simulink model "MSDR_v1"  (R2018a)
settings: Solver=ode23tb  StartTime=0.0  StopTime=50000  RelTol=1e-3
values from neighbouring files (symbols this model uses):
  a_f = -3.22E-5    (= -3.22e-05)    [MSDR_parameters.m]
  a_g = +2.35E-5    (= 2.35e-05)    [MSDR_parameters.m]
  beta = [0.000223, 0.001457, 0.001307, 0.002628, 0.000766, 0.000280]    [MSDR_parameters.m]
  beta_t = sum(beta)    [MSDR_parameters.m]
  Cp_s_shx = 1549.12e-6    (= 0.00154912)    [MSDR_parameters.m]
  Cst = 10    [MSDR_parameters.m]
  dLb = 0    [MSDR_parameters.m]
  dLs = 0    [MSDR_parameters.m]
  dLsc = 0    [MSDR_parameters.m]
  gamma_I = 5.1135e-2    (= 0.051135)    [MSDR_parameters.m]
  gamma_Xe = 1.1628e-2    (= 0.011628)    [MSDR_parameters.m]
  hA_fg = [h_fg*A_fg/2, h_fg*A_fg/2]    [MSDR_parameters.m]
  hA_p_phx1 = h_p_phx*A_p_phx    [MSDR_parameters.m]
  hA_p_phx2 = h_p_phx*A_p_phx    [MSDR_parameters.m]
  hA_p_phx3 = h_p_phx*A_p_phx    [MSDR_parameters.m]
  hA_p_phx4 = h_p_phx*A_p_phx    [MSDR_parameters.m]
  hA_p_phx5 = h_p_phx*A_p_phx    [MSDR_parameters.m]
  hA_p_phx6 = h_p_phx*A_p_phx    [MSDR_parameters.m]
  hA_p_shx1 = h_p_shx*A_p_shx    [MSDR_parameters.m]
  hA_p_shx2 = h_p_shx*A_p_shx    [MSDR_parameters.m]
  hA_p_shx3 = h_p_shx*A_p_shx    [MSDR_parameters.m]
  hA_p_shx4 = h_p_shx*A_p_shx    [MSDR_parameters.m]
  hA_p_shx5 = h_p_shx*A_p_shx    [MSDR_parameters.m]
  hA_p_shx6 = h_p_shx*A_p_shx    [MSDR_parameters.m]
  hA_s_phx1 = h_s_phx*A_s_phx    [MSDR_parameters.m]
  hA_s_phx2 = h_s_phx*A_s_phx    [MSDR_parameters.m]
  hA_s_phx3 = h_s_phx*A_s_phx    [MSDR_parameters.m]
  hA_s_phx4 = h_s_phx*A_s_phx    [MSDR_parameters.m]
  hA_s_phx5 = h_s_phx*A_s_phx    [MSDR_parameters.m]
  hA_s_phx6 = h_s_phx*A_s_phx    [MSDR_parameters.m]
  hA_s_shx1 = h_s_shx*A_s_shx    [MSDR_parameters.m]
  hA_s_shx2 = h_s_shx*A_s_shx    [MSDR_parameters.m]
  hA_s_shx3 = h_s_shx*A_s_shx    [MSDR_parameters.m]
  hA_s_shx4 = h_s_shx*A_s_shx    [MSDR_parameters.m]
  hA_s_shx5 = h_s_shx*A_s_shx    [MSDR_parameters.m]
  hA_s_shx6 = h_s_shx*A_s_shx    [MSDR_parameters.m]
  I_0 = gamma_I*Sig_f_msdr*phi_0/lam_I    (= 4.38204721773e+16)    [MSDR_parameters.m]
  Ifa = [0.25, 0.25]    [MSDR_parameters.m]
  Ifb = [0.25, 0.25]    [MSDR_parameters.m]
  Ig = [0.5, 0.5]    [MSDR_parameters.m]
  J = 1e-6    (= 1e-06)    [MSDR_parameters.m]
  ka = [0.235, 0.235]    [MSDR_parameters.m]
  kb = [0.235, 0.235]    [MSDR_parameters.m]
  kc = 5    [MSDR_parameters.m]
  kga = [0.015, 0.015]    [MSDR_parameters.m]
  kgb = [0.015, 0.015]    [MSDR_parameters.m]
  L = 8.5344    [MSDR_parameters.m]
  Lam = 2.400E-04    (= 0.00024)    [MSDR_parameters.m]
  lam = [0.0124, 0.0305, 0.111, 0.301, 1.14, 3.01]    [MSDR_parameters.m]
  lam_bubl = 2.0e-2    (= 0.02)    [MSDR_parameters.m]
  lam_I = 2.875e-5    (= 2.875e-05)    [MSDR_parameters.m]
  lam_Xe = 2.0916e-5    (= 2.0916e-05)    [MSDR_parameters.m]
  m_3m = W_3*2    (= 8618.207327)    [MSDR_parameters.m]
  m_fm = W_f*2    (= 9978.96)    [MSDR_parameters.m]
  m_sb = 1717    [MSDR_parameters.m]
  mb_cpb = 2.689619410657651e+00    (= 2.68961941066)    [MSDR_parameters.m]
  mcp_fa = mfa*Cp_f    [MSDR_parameters.m]
  mcp_fb = mfb*Cp_f    [MSDR_parameters.m]
  mcp_g = mg*Cp_g    [MSDR_parameters.m]
  mcp_p_phx1 = Cp_p_phx*mp_phx1    [MSDR_parameters.m]
  mcp_p_phx2 = Cp_p_phx*mp_phx2    [MSDR_parameters.m]
  mcp_p_phx3 = Cp_p_phx*mp_phx3    [MSDR_parameters.m]
  mcp_p_phx4 = Cp_p_phx*mp_phx4    [MSDR_parameters.m]
  mcp_p_phx5 = Cp_p_phx*mp_phx5    [MSDR_parameters.m]
  mcp_p_phx6 = Cp_p_phx*mp_phx6    [MSDR_parameters.m]
  mcp_p_shx1 = Cp_p_shx*mp_shx1    [MSDR_parameters.m]
  mcp_p_shx2 = Cp_p_shx*mp_shx2    [MSDR_parameters.m]
  mcp_p_shx3 = Cp_p_shx*mp_shx3    [MSDR_parameters.m]
  mcp_p_shx4 = Cp_p_shx*mp_shx4    [MSDR_parameters.m]
  mcp_p_shx5 = Cp_p_shx*mp_shx5    [MSDR_parameters.m]
  mcp_p_shx6 = Cp_p_shx*mp_shx6    [MSDR_parameters.m]
  mcp_s_phx1 = Cp_s_phx*ms_phx1    [MSDR_parameters.m]
  mcp_s_phx2 = Cp_s_phx*ms_phx2    [MSDR_parameters.m]
  mcp_s_phx3 = Cp_s_phx*ms_phx3    [MSDR_parameters.m]
  mcp_s_phx4 = Cp_s_phx*ms_phx4    [MSDR_parameters.m]
  mcp_s_phx5 = Cp_s_phx*ms_phx5    [MSDR_parameters.m]
  mcp_s_phx6 = Cp_s_phx*ms_phx6    [MSDR_parameters.m]
  mcp_s_shx1 = Cp_s_shx*ms_shx1    [MSDR_parameters.m]
  mcp_s_shx2 = Cp_s_shx*ms_shx1    [MSDR_parameters.m]
  mcp_s_shx3 = Cp_s_shx*ms_shx1    [MSDR_parameters.m]
  mcp_s_shx4 = Cp_s_shx*ms_shx1    [MSDR_parameters.m]
  mcp_s_shx5 = Cp_s_shx*ms_shx1    [MSDR_parameters.m]
  mcp_s_shx6 = Cp_s_shx*ms_shx1    [MSDR_parameters.m]
  mcp_t_phx1 = Cp_t_phx*mt_phx1    [MSDR_parameters.m]
  mcp_t_phx2 = Cp_t_phx*mt_phx2    [MSDR_parameters.m]
  mcp_t_phx3 = Cp_t_phx*mt_phx3    [MSDR_parameters.m]
  mcp_t_phx4 = Cp_t_phx*mt_phx4    [MSDR_parameters.m]
  mcp_t_phx5 = Cp_t_phx*mt_phx5    [MSDR_parameters.m]
  mcp_t_phx6 = Cp_t_phx*mt_phx6    [MSDR_parameters.m]
  mcp_t_shx1 = Cp_t_phx*mt_shx1    [MSDR_parameters.m]
  mcp_t_shx2 = Cp_t_phx*mt_shx2    [MSDR_parameters.m]
  mcp_t_shx3 = Cp_t_phx*mt_shx3    [MSDR_parameters.m]
  mcp_t_shx4 = Cp_t_phx*mt_shx4    [MSDR_parameters.m]
  mcp_t_shx5 = Cp_t_phx*mt_shx5    [MSDR_parameters.m]
  mcp_t_shx6 = Cp_t_phx*mt_shx6    [MSDR_parameters.m]
  mfa = [mass_fn, mass_fn]    [MSDR_parameters.m]
  mfb = [mass_fn, mass_fn]    [MSDR_parameters.m]
  mp_phx1 = [494.7, 494.7, 494.7, 494.7]    [MSDR_parameters.m]
  mp_phx2 = [494.7, 494.7, 494.7, 494.7]    [MSDR_parameters.m]
  mp_phx3 = [494.7, 494.7, 494.7, 494.7]    [MSDR_parameters.m]
  mp_phx4 = [494.7, 494.7, 494.7, 494.7]    [MSDR_parameters.m]
  mp_phx5 = [494.7, 494.7, 494.7, 494.7]    [MSDR_parameters.m]
  mp_phx6 = [494.7, 494.7, 494.7, 494.7]    [MSDR_parameters.m]
  mp_phxm = (Wp_phx1 + Wp_phx2)*1    (= 1663.16)    [MSDR_parameters.m]
  mp_shx1 = [429.3, 429.3, 429.3, 429.3]    [MSDR_parameters.m]
  mp_shx2 = [429.3, 429.3, 429.3, 429.3]    [MSDR_parameters.m]
  mp_shx3 = [429.3, 429.3, 429.3, 429.3]    [MSDR_parameters.m]
  mp_shx4 = [429.3, 429.3, 429.3, 429.3]    [MSDR_parameters.m]
  mp_shx5 = [429.3, 429.3, 429.3, 429.3]    [MSDR_parameters.m]
  mp_shx6 = [429.3, 429.3, 429.3, 429.3]    [MSDR_parameters.m]
  mp_shxm = (Wp_shx1 + Wp_shx2)*1    (= 932.38)    [MSDR_parameters.m]
  ms_phx1 = [1152.5, 1152.5, 1152.5, 1152.5]    [MSDR_parameters.m]
  ms_phx2 = [1152.5, 1152.5, 1152.5, 1152.5]    [MSDR_parameters.m]
  ms_phx3 = [1152.5, 1152.5, 1152.5, 1152.5]    [MSDR_parameters.m]
  ms_phx4 = [1152.5, 1152.5, 1152.5, 1152.5]    [MSDR_parameters.m]
  ms_phx5 = [1152.5, 1152.5, 1152.5, 1152.5]    [MSDR_parameters.m]
  ms_phx6 = [1152.5, 1152.5, 1152.5, 1152.5]    [MSDR_parameters.m]
  ms_phxm = (Ws_phx1 + Ws_phx2)*1    (= 932.38)    [MSDR_parameters.m]
  ms_shx1 = [1861.5, 1861.5, 1861.5, 1861.5]    [MSDR_parameters.m]
  ms_shx2 = [1861.5, 1861.5, 1861.5, 1861.5]    [MSDR_parameters.m]
  ... (+104 more)
undefined symbols (not defined in the file or in its folder): Ak2, As, C0, Cpp, Cps, Cpsc, Cpw, Dit, Dot, hA_p_thx1, hA_p_thx2, hA_p_thx3, hA_s_thx1, hA_s_thx2, hA_s_thx3, hc0, hfg, hfw0, HFW1, hfw10, HFW2, hpw, Hr, hr0, hwb, hws, hwsc, K3, KBHP, KBLP, Lsc, mcp_p_thx1, mcp_p_thx2, mcp_p_thx3, mcp_s_thx1, mcp_s_thx2, mcp_s_thx3, mcp_t_thx1, mcp_t_thx2, mcp_t_thx3, mp_thx1, mp_thx2, mp_thx3, ms_thx1, ms_thx2, ms_thx3, Mstm, nuf, Pp2, Pp3, Pp4, Pp5
libraries: simulink x20, aerolibconvert2 x2
(part 2 of 7)

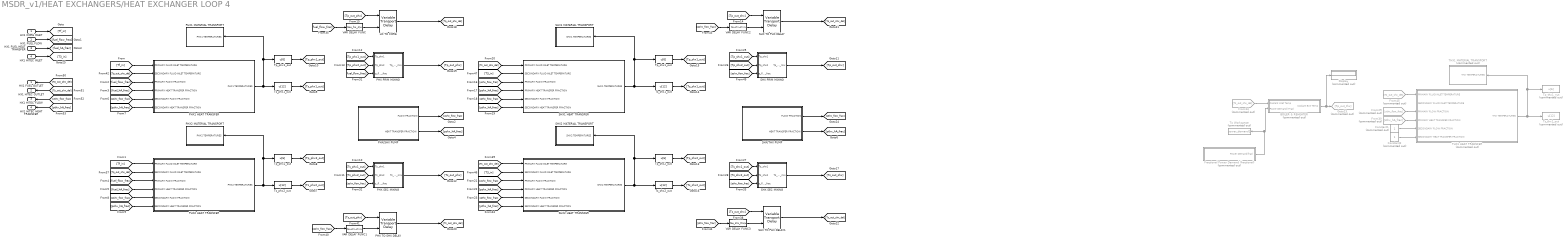
== system MSDR_v1/HEAT EXCHANGERS/HEAT EXCHANGER LOOP 4 ==
  HX1 CORE INLET : Inport
  HX1 FUEL FLOW : Inport  Port=2
  HX1 FUEL HEAT TRANSFER : Inport  Port=3
  HX1 HITEC INLET : Inport  Port=4
  BOILER & REHEATER : Subsystem  Commented=on
  Constant1 : Constant  Commented=on
  Constant2 : Constant  Commented=on
  Display : Display  Commented=on
  Fractional Power Demand (fractional) : Subsystem  Commented=on
  From29 : From  Commented=on  GotoTag=sthx_flow_frac
  From30 : From  Commented=on  GotoTag=sthx_hA_frac
  From34 : From  Commented=on  GotoTag=Ts_out_shx_del
  From45 : From  Commented=on  GotoTag=Ts_out_shx_del
  Goto23 : Goto  Commented=on  GotoTag=Tp_out_thx
  HX TO CORE : VariableTransportDelay  MaximumDelay=1000000000000  InitialOutput=T0_p_phx1(4)
  PHX PRIM MIXING : Subsystem
  PHX SEC MIXING : Subsystem
  PHX TO SHX DELAY : VariableTransportDelay  MaximumDelay=100000000000  InitialOutput=T0_s_phx1(4)
  PHX/SHX PUMP : Subsystem
  PHX1 HEAT TRANSFER : Subsystem
  PHX1 MATERIAL TRANSPORT : Subsystem
  PHX2 HEAT TRANSFER : Subsystem
  PHX2 MATERIAL TRANSPORT : Subsystem
  SHX PRIM MIXING : Subsystem
  SHX SEC MIXING : Subsystem
  SHX TO PHX DELAY : VariableTransportDelay  MaximumDelay=1000000000000  InitialOutput=T0_p_shx1(4)
  SHX TO PHX DELAY1 : VariableTransportDelay  MaximumDelay=1000000000000  InitialOutput=T0_s_shx1(4)
  SHX/THX PUMP : Subsystem
  SHX1 HEAT TRANSFER : Subsystem
  SHX1 MATERIAL TRANSPORT : Subsystem
  SHX2 HEAT TRANSFER : Subsystem
  SHX2 MATERIAL TRANSPORT : Subsystem
  THX1 HEAT TRANSFER : Subsystem  Commented=on
  THX1 MATERIAL TRANSPORT : Subsystem  Commented=on
  To Workspace : ToWorkspace  Commented=on  VariableName=power_demand1  SampleTime=-1
  Tp_phx1_out : Fcn  Expr=u[6]
  Tp_phx2_out : Fcn  Expr=u[6]
  Tp_shx1_out : Fcn  Expr=u[6]
  Tp_shx2_out : Fcn  Expr=u[6]
  Tp_thx1_out : Fcn  Commented=on  Expr=u[6]
  Ts_phx1_out : Fcn  Expr=u[12]
  Ts_phx2_out : Fcn  Expr=u[12]
  Ts_shx1_out : Fcn  Expr=u[12]
  Ts_shx2_out : Fcn  Expr=u[12]
  Ts_thx1_out : Fcn  Commented=on  Expr=u[12]
  VAR DELAY FUNC : Fcn  Expr=tau_hx_c/u
  VAR DELAY FUNC1 : Fcn  Expr=tau_phx_shx/u
  VAR DELAY FUNC2 : Fcn  Expr=tau_shx_phx/u
  VAR DELAY FUNC3 : Fcn  Expr=tau_shx_thx/u
  HX1 FUEL OUTLET : Outport
  HX1 HITEC OUTLET : Outport  Port=2
  HX1 HITEC FLOW : Outport  Port=3
  HX1 HITEC HEAT TRANSFER : Outport  Port=4
  wires:
  PHX1 HEAT TRANSFER/1(PHX1 TEMPERATURES) -> PHX1 MATERIAL TRANSPORT/1(PHX1 TEMPERATURES), Tp_phx1_out/1, Ts_phx1_out/1
  THX1 HEAT TRANSFER/1(THX TEMPERATURES) -> THX1 MATERIAL TRANSPORT/1(THX TEMPERATURES), Tp_thx1_out/1, Ts_thx1_out/1
  SHX1 HEAT TRANSFER/1(SHX1 TEMPERATURES) -> Ts_shx1_out/1, Tp_shx1_out/1, SHX1 MATERIAL TRANSPORT/1(SHX1 TEMPERATURES)
  PHX2 HEAT TRANSFER/1(PHX2 TEMPERATURES) -> PHX2 MATERIAL TRANSPORT/1(PHX2 TEMPERATURES), Tp_phx2_out/1, Ts_phx2_out/1
  SHX2 HEAT TRANSFER/1(SHX2 TEMPERATURES) -> Ts_shx2_out/1, SHX2 MATERIAL TRANSPORT/1(SHX2 TEMPERATURES), Tp_shx2_out/1
  HX1 CORE INLET/1 -> [Tf_in]
  [Tf_in] -> PHX1 HEAT TRANSFER/1(PRIMARY FLUID INLET TEMPERATURE)
  [Tf_in] -> PHX2 HEAT TRANSFER/1(PRIMARY FLUID INLET TEMPERATURE)
  HX1 FUEL FLOW/1 -> [fuel_flow_frac]
  HX1 FUEL HEAT TRANSFER/1 -> [fuel_hA_frac]
  [fuel_flow_frac] -> PHX1 HEAT TRANSFER/3(PRIMARY FLOW FRACTION)
  [fuel_hA_frac] -> PHX1 HEAT TRANSFER/4(PRIMARY HEAT TRANSFER FRACTION)
  [fuel_flow_frac] -> PHX2 HEAT TRANSFER/3(PRIMARY FLOW FRACTION)
  [fuel_hA_frac] -> PHX2 HEAT TRANSFER/4(PRIMARY HEAT TRANSFER FRACTION)
  PHX/SHX PUMP/2(HEAT TRANSFER FRACTION) -> [pshx_hA_frac]
  PHX/SHX PUMP/1(FLOW FRACTION) -> [pshx_flow_frac]
  SHX/THX PUMP/1(FLOW FRACTION) -> [pthx_flow_frac]
  SHX/THX PUMP/2(HEAT TRANSFER FRACTION) -> [pthx_hA_frac]
  Ts_phx2_out/1 -> [Ts_phx2_out]
  Tp_phx2_out/1 -> [Tp_phx2_out]
  Tp_phx1_out/1 -> [Tp_phx1_out]
  Ts_phx1_out/1 -> [Ts_phx1_out]
  [pshx_flow_frac] -> PHX1 HEAT TRANSFER/5(SECONDARY FLOW FRACTION)
  [pshx_hA_frac] -> PHX1 HEAT TRANSFER/6(SECONDARY HEAT TRANSFER FRACTION)
  [pshx_flow_frac] -> PHX2 HEAT TRANSFER/5(SECONDARY FLOW FRACTION)
  [pshx_hA_frac] -> PHX2 HEAT TRANSFER/6(SECONDARY HEAT TRANSFER FRACTION)
  [Tp_phx1_out] -> PHX PRIM MIXING/1(Tp_phx1)
  [Tp_phx2_out] -> PHX PRIM MIXING/2(Tp_phx2)
  PHX PRIM MIXING/1(Tp_phx_mix) -> [Tp_out_phx]
  [Ts_out_phx_del] -> SHX1 HEAT TRANSFER/1(PRIMARY FLUID INLET TEMPERATURE)
  [pshx_flow_frac] -> SHX1 HEAT TRANSFER/3(PRIMARY FLOW FRACTION)
  [pshx_hA_frac] -> SHX1 HEAT TRANSFER/4(PRIMARY HEAT TRANSFER FRACTION)
  [pthx_flow_frac] -> SHX1 HEAT TRANSFER/5(SECONDARY FLOW FRACTION)
  [pthx_hA_frac] -> SHX1 HEAT TRANSFER/6(SECONDARY HEAT TRANSFER FRACTION)
  [Ts_out_phx_del] -> SHX2 HEAT TRANSFER/1(PRIMARY FLUID INLET TEMPERATURE)
  [pshx_flow_frac] -> SHX2 HEAT TRANSFER/3(PRIMARY FLOW FRACTION)
  [pshx_hA_frac] -> SHX2 HEAT TRANSFER/4(PRIMARY HEAT TRANSFER FRACTION)
  [pthx_flow_frac] -> SHX2 HEAT TRANSFER/5(SECONDARY FLOW FRACTION)
  [pthx_hA_frac] -> SHX2 HEAT TRANSFER/6(SECONDARY HEAT TRANSFER FRACTION)
  Tp_shx1_out/1 -> [Tp_shx1_out]
  Tp_shx2_out/1 -> [Tp_shx2_out]
  Ts_shx1_out/1 -> [Ts_shx1_out]
  Ts_shx2_out/1 -> [Ts_shx2_out]
  From29/1 -> THX1 HEAT TRANSFER/3(PRIMARY FLOW FRACTION)
  From30/1 -> THX1 HEAT TRANSFER/4(PRIMARY HEAT TRANSFER FRACTION)
  [fuel_flow_frac] -> PHX PRIM MIXING/3(p_flow_frac)
  [pshx_flow_frac] -> PHX SEC MIXING/3(s_flow_frac)
  [Ts_phx2_out] -> PHX SEC MIXING/2(Ts_phx2)
  [Ts_phx1_out] -> PHX SEC MIXING/1(Ts_phx1)
  PHX SEC MIXING/1(Ts_phx_mix) -> [Ts_out_phx]
  [Tp_shx2_out] -> SHX PRIM MIXING/2(Tp_shx2)
  [Tp_shx1_out] -> SHX PRIM MIXING/1(Tp_shx1)
  SHX PRIM MIXING/1(Tp_shx_mix) -> [Tp_out_shx]
  From45/1 -> THX1 HEAT TRANSFER/1(PRIMARY FLUID INLET TEMPERATURE)
  [Ts_shx1_out] -> SHX SEC MIXING/1(Ts_shx1)
  SHX SEC MIXING/1(Ts_shx_mix) -> [Ts_out_shx]
  [Ts_shx2_out] -> SHX SEC MIXING/2(Ts_shx2)
  [pthx_flow_frac] -> SHX SEC MIXING/3(s_flow_frac)
  Constant1/1 -> THX1 HEAT TRANSFER/5(SECONDARY FLOW FRACTION)
  Constant2/1 -> THX1 HEAT TRANSFER/6(SECONDARY HEAT TRANSFER FRACTION)
  [Tp_out_shx_del] -> PHX1 HEAT TRANSFER/2(SECONDARY FLUID INLET TEMPERATURE)
  [Tp_out_shx_del] -> PHX2 HEAT TRANSFER/2(SECONDARY FLUID INLET TEMPERATURE)
  VAR DELAY FUNC/1 -> HX TO CORE/2
  [Tp_out_phx] -> HX TO CORE/1
  [fuel_flow_frac] -> VAR DELAY FUNC/1
  HX TO CORE/1 -> [Tp_out_phx_del]
  VAR DELAY FUNC1/1 -> PHX TO SHX DELAY/2
  PHX TO SHX DELAY/1 -> [Ts_out_phx_del]
  [Ts_out_phx] -> PHX TO SHX DELAY/1
  [pshx_flow_frac] -> VAR DELAY FUNC1/1
  VAR DELAY FUNC2/1 -> SHX TO PHX DELAY/2
  SHX TO PHX DELAY/1 -> [Tp_out_shx_del]
  [pshx_flow_frac] -> VAR DELAY FUNC2/1
  [Tp_out_shx] -> SHX TO PHX DELAY/1
  [Ts_out_shx] -> SHX TO PHX DELAY1/1
  [pthx_flow_frac] -> VAR DELAY FUNC3/1
  SHX TO PHX DELAY1/1 -> [Ts_out_shx_del]
  VAR DELAY FUNC3/1 -> SHX TO PHX DELAY1/2
  Fractional Power Demand (fractional)/1(Power Demand(frac)) -> BOILER & REHEATER/2(Power Demand (Frac)), To Workspace/1
  From34/1 -> BOILER & REHEATER/1(Coolant Inlet Temp)
  BOILER & REHEATER/1(Coolant Exit Temp) -> Display/1, Goto23/1
  [T3_in] -> SHX1 HEAT TRANSFER/2(SECONDARY FLUID INLET TEMPERATURE)
  [T3_in] -> SHX2 HEAT TRANSFER/2(SECONDARY FLUID INLET TEMPERATURE)
  HX1 HITEC INLET/1 -> [T3_in]
  [pshx_flow_frac] -> SHX PRIM MIXING/3(p_flow_frac)
  [pthx_hA_frac] -> HX1 HITEC HEAT TRANSFER/1
  [pthx_flow_frac] -> HX1 HITEC FLOW/1
  [Ts_out_shx_del] -> HX1 HITEC OUTLET/1
  [Tp_out_phx_del] -> HX1 FUEL OUTLET/1

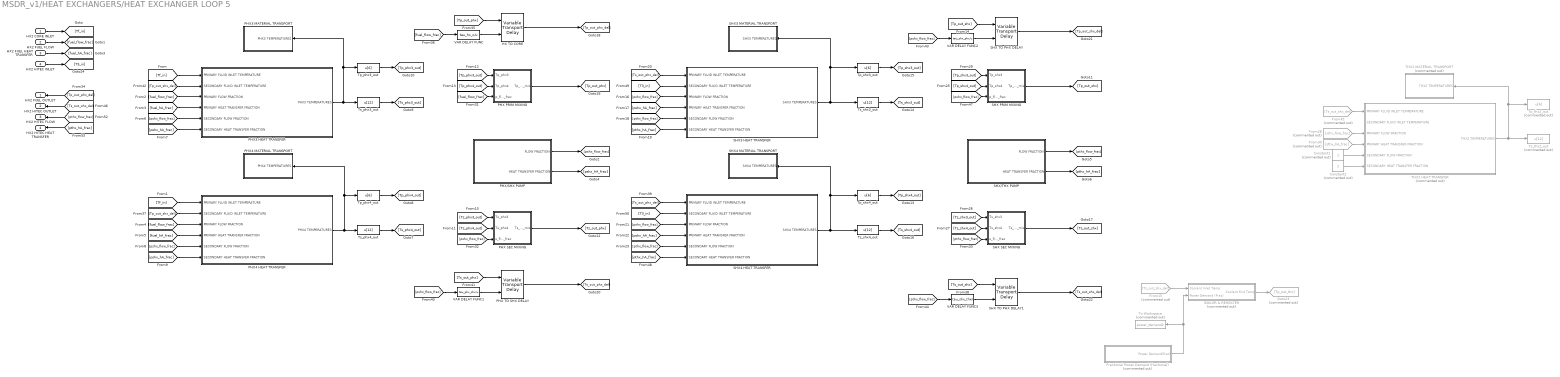
== system MSDR_v1/HEAT EXCHANGERS/HEAT EXCHANGER LOOP 5 ==
  HX2 CORE INLET : Inport
  HX2 FUEL FLOW : Inport  Port=2
  HX2 FUEL HEAT TRANSFER : Inport  Port=3
  HX2 HITEC INLET : Inport  Port=4
  BOILER & REHEATER : Subsystem  Commented=on
  Constant1 : Constant  Commented=on
  Constant2 : Constant  Commented=on
  Fractional Power Demand (fractional) : Subsystem  Commented=on
  From15 : From  Commented=on  GotoTag=Ts_out_shx_del
  From28 : From  Commented=on  GotoTag=sthx_flow_frac
  From30 : From  Commented=on  GotoTag=sthx_hA_frac
  From45 : From  Commented=on  GotoTag=Ts_out_shx_del
  Goto23 : Goto  Commented=on  GotoTag=Tp_out_thx
  HX TO CORE : VariableTransportDelay  MaximumDelay=1000000000000  InitialOutput=T0_p_phx3(4)
  PHX PRIM MIXING : Subsystem
  PHX SEC MIXING : Subsystem
  PHX TO SHX DELAY : VariableTransportDelay  MaximumDelay=100000000000  InitialOutput=T0_s_phx3(4)
  PHX/SHX PUMP : Subsystem
  PHX3 HEAT TRANSFER : Subsystem
  PHX3 MATERIAL TRANSPORT : Subsystem
  PHX4 HEAT TRANSFER : Subsystem
  PHX4 MATERIAL TRANSPORT : Subsystem
  SHX PRIM MIXING : Subsystem
  SHX SEC MIXING : Subsystem
  SHX TO PHX DELAY : VariableTransportDelay  MaximumDelay=1000000000000  InitialOutput=T0_p_shx3(4)
  SHX TO PHX DELAY1 : VariableTransportDelay  MaximumDelay=1000000000000  InitialOutput=T0_s_shx3(4)
  SHX/THX PUMP : Subsystem
  SHX3 HEAT TRANSFER : Subsystem
  SHX3 MATERIAL TRANSPORT : Subsystem
  SHX4 HEAT TRANSFER : Subsystem
  SHX4 MATERIAL TRANSPORT : Subsystem
  THX2 HEAT TRANSFER : Subsystem  Commented=on
  THX2 MATERIAL TRANSPORT : Subsystem  Commented=on
  To Workspace : ToWorkspace  Commented=on  VariableName=power_demand2  SampleTime=-1
  Tp_phx3_out : Fcn  Expr=u[6]
  Tp_phx4_out : Fcn  Expr=u[6]
  Tp_shx3_out : Fcn  Expr=u[6]
  Tp_shx4_out : Fcn  Expr=u[6]
  Tp_thx2_out : Fcn  Commented=on  Expr=u[6]
  Ts_phx3_out : Fcn  Expr=u[12]
  Ts_phx4_out : Fcn  Expr=u[12]
  Ts_shx3_out : Fcn  Expr=u[12]
  Ts_shx4_out : Fcn  Expr=u[12]
  Ts_thx2_out : Fcn  Commented=on  Expr=u[12]
  VAR DELAY FUNC : Fcn  Expr=tau_hx_c/u
  VAR DELAY FUNC1 : Fcn  Expr=tau_phx_shx/u
  VAR DELAY FUNC2 : Fcn  Expr=tau_shx_phx/u
  VAR DELAY FUNC3 : Fcn  Expr=tau_shx_thx/u
  HX2 FUEL OUTLET : Outport
  HX2 HITEC OUTLET : Outport  Port=2
  HX2 HITEC FLOW : Outport  Port=3
  HX2 HITEC HEAT TRANSFER : Outport  Port=4
  wires:
  [Tp_out_phx_del] -> HX2 FUEL OUTLET/1
  HX2 CORE INLET/1 -> [Tf_in]
  HX2 FUEL HEAT TRANSFER/1 -> [fuel_hA_frac]
  HX2 FUEL FLOW/1 -> [fuel_flow_frac]
  Tp_phx3_out/1 -> [Tp_phx3_out]
  PHX3 HEAT TRANSFER/1(PHX3 TEMPERATURES) -> PHX3 MATERIAL TRANSPORT/1(PHX3 TEMPERATURES), Tp_phx3_out/1, Ts_phx3_out/1
  Ts_phx3_out/1 -> [Ts_phx3_out]
  Tp_phx4_out/1 -> [Tp_phx4_out]
  Ts_phx4_out/1 -> [Ts_phx4_out]
  PHX4 HEAT TRANSFER/1(PHX4 TEMPERATURES) -> PHX4 MATERIAL TRANSPORT/1(PHX4 TEMPERATURES), Tp_phx4_out/1, Ts_phx4_out/1
  Tp_shx3_out/1 -> [Tp_shx3_out]
  Ts_shx3_out/1 -> [Ts_shx3_out]
  SHX3 HEAT TRANSFER/1(SHX3 TEMPERATURES) -> Ts_shx3_out/1, SHX3 MATERIAL TRANSPORT/1(SHX3 TEMPERATURES), Tp_shx3_out/1
  [Tp_phx3_out] -> PHX PRIM MIXING/1(Tp_phx3)
  [fuel_flow_frac] -> PHX PRIM MIXING/3(p_flow_frac)
  [Ts_phx3_out] -> PHX SEC MIXING/1(Ts_phx3)
  [Ts_phx4_out] -> PHX SEC MIXING/2(Ts_phx4)
  [Tp_phx4_out] -> PHX PRIM MIXING/2(Tp_phx4)
  PHX SEC MIXING/1(Ts_phx_mix) -> [Ts_out_phx]
  PHX/SHX PUMP/1(FLOW FRACTION) -> [pshx_flow_frac]
  PHX PRIM MIXING/1(Tp_phx_mix) -> [Tp_out_phx]
  [pshx_flow_frac] -> PHX SEC MIXING/3(s_flow_frac)
  PHX/SHX PUMP/2(HEAT TRANSFER FRACTION) -> [pshx_hA_frac]
  Tp_shx4_out/1 -> [Tp_shx4_out]
  SHX4 HEAT TRANSFER/1(SHX4 TEMPERATURES) -> Ts_shx4_out/1, SHX4 MATERIAL TRANSPORT/1(SHX4 TEMPERATURES), Tp_shx4_out/1
  Ts_shx4_out/1 -> [Ts_shx4_out]
  [Tp_shx3_out] -> SHX PRIM MIXING/1(Tp_shx3)
  [Ts_shx4_out] -> SHX SEC MIXING/2(Ts_shx4)
  [Ts_shx3_out] -> SHX SEC MIXING/1(Ts_shx3)
  [Tp_shx4_out] -> SHX PRIM MIXING/2(Tp_shx4)
  SHX/THX PUMP/2(HEAT TRANSFER FRACTION) -> [pthx_hA_frac]
  SHX SEC MIXING/1(Ts_shx_mix) -> [Ts_out_shx]
  SHX PRIM MIXING/1(Tp_shx_mix) -> [Tp_out_shx]
  SHX/THX PUMP/1(FLOW FRACTION) -> [pthx_flow_frac]
  [pthx_flow_frac] -> SHX SEC MIXING/3(s_flow_frac)
  THX2 HEAT TRANSFER/1(THX2 TEMPERATURES) -> THX2 MATERIAL TRANSPORT/1(THX2 TEMPERATURES), Tp_thx2_out/1, Ts_thx2_out/1
  [fuel_hA_frac] -> PHX3 HEAT TRANSFER/4(PRIMARY HEAT TRANSFER FRACTION)
  [Tp_out_shx_del] -> PHX3 HEAT TRANSFER/2(SECONDARY FLUID INLET TEMPERATURE)
  [pshx_hA_frac] -> PHX3 HEAT TRANSFER/6(SECONDARY HEAT TRANSFER FRACTION)
  [Tf_in] -> PHX3 HEAT TRANSFER/1(PRIMARY FLUID INLET TEMPERATURE)
  [pshx_flow_frac] -> PHX3 HEAT TRANSFER/5(SECONDARY FLOW FRACTION)
  [fuel_flow_frac] -> PHX3 HEAT TRANSFER/3(PRIMARY FLOW FRACTION)
  [Tp_out_shx_del] -> PHX4 HEAT TRANSFER/2(SECONDARY FLUID INLET TEMPERATURE)
  [pshx_flow_frac] -> PHX4 HEAT TRANSFER/5(SECONDARY FLOW FRACTION)
  [fuel_flow_frac] -> PHX4 HEAT TRANSFER/3(PRIMARY FLOW FRACTION)
  [Tf_in] -> PHX4 HEAT TRANSFER/1(PRIMARY FLUID INLET TEMPERATURE)
  [pshx_hA_frac] -> PHX4 HEAT TRANSFER/6(SECONDARY HEAT TRANSFER FRACTION)
  [fuel_hA_frac] -> PHX4 HEAT TRANSFER/4(PRIMARY HEAT TRANSFER FRACTION)
  VAR DELAY FUNC/1 -> HX TO CORE/2
  HX TO CORE/1 -> [Tp_out_phx_del]
  [Tp_out_phx] -> HX TO CORE/1
  [fuel_flow_frac] -> VAR DELAY FUNC/1
  [Ts_out_phx] -> PHX TO SHX DELAY/1
  [pshx_flow_frac] -> VAR DELAY FUNC1/1
  VAR DELAY FUNC1/1 -> PHX TO SHX DELAY/2
  PHX TO SHX DELAY/1 -> [Ts_out_phx_del]
  [pthx_flow_frac] -> SHX3 HEAT TRANSFER/5(SECONDARY FLOW FRACTION)
  [pthx_hA_frac] -> SHX3 HEAT TRANSFER/6(SECONDARY HEAT TRANSFER FRACTION)
  [pshx_hA_frac] -> SHX3 HEAT TRANSFER/4(PRIMARY HEAT TRANSFER FRACTION)
  [Ts_out_phx_del] -> SHX3 HEAT TRANSFER/1(PRIMARY FLUID INLET TEMPERATURE)
  [pshx_flow_frac] -> SHX3 HEAT TRANSFER/3(PRIMARY FLOW FRACTION)
  [pthx_hA_frac] -> SHX4 HEAT TRANSFER/6(SECONDARY HEAT TRANSFER FRACTION)
  [pthx_flow_frac] -> SHX4 HEAT TRANSFER/5(SECONDARY FLOW FRACTION)
  [pshx_hA_frac] -> SHX4 HEAT TRANSFER/4(PRIMARY HEAT TRANSFER FRACTION)
  [pshx_flow_frac] -> SHX4 HEAT TRANSFER/3(PRIMARY FLOW FRACTION)
  [Ts_out_phx_del] -> SHX4 HEAT TRANSFER/1(PRIMARY FLUID INLET TEMPERATURE)
  [Tp_out_shx] -> SHX TO PHX DELAY/1
  [pshx_flow_frac] -> VAR DELAY FUNC2/1
  SHX TO PHX DELAY/1 -> [Tp_out_shx_del]
  VAR DELAY FUNC2/1 -> SHX TO PHX DELAY/2
  VAR DELAY FUNC3/1 -> SHX TO PHX DELAY1/2
  SHX TO PHX DELAY1/1 -> [Ts_out_shx_del]
  [Ts_out_shx] -> SHX TO PHX DELAY1/1
  [pthx_flow_frac] -> VAR DELAY FUNC3/1
  From30/1 -> THX2 HEAT TRANSFER/4(PRIMARY HEAT TRANSFER FRACTION)
  From45/1 -> THX2 HEAT TRANSFER/1(PRIMARY FLUID INLET TEMPERATURE)
  Constant1/1 -> THX2 HEAT TRANSFER/5(SECONDARY FLOW FRACTION)
  Constant2/1 -> THX2 HEAT TRANSFER/6(SECONDARY HEAT TRANSFER FRACTION)
  From28/1 -> THX2 HEAT TRANSFER/3(PRIMARY FLOW FRACTION)
  BOILER & REHEATER/1(Coolant Exit Temp) -> Goto23/1
  From15/1 -> BOILER & REHEATER/1(Coolant Inlet Temp)
  Fractional Power Demand (fractional)/1(Power Demand(frac)) -> BOILER & REHEATER/2(Power Demand (Frac)), To Workspace/1
  [T3_in] -> SHX3 HEAT TRANSFER/2(SECONDARY FLUID INLET TEMPERATURE)
  [T3_in] -> SHX4 HEAT TRANSFER/2(SECONDARY FLUID INLET TEMPERATURE)
  HX2 HITEC INLET/1 -> [T3_in]
  [Ts_out_shx_del] -> HX2 HITEC OUTLET/1
  [pshx_flow_frac] -> SHX PRIM MIXING/3(p_flow_frac)
  [pthx_flow_frac] -> HX2 HITEC FLOW/1
  [pthx_hA_frac] -> HX2 HITEC HEAT TRANSFER/1

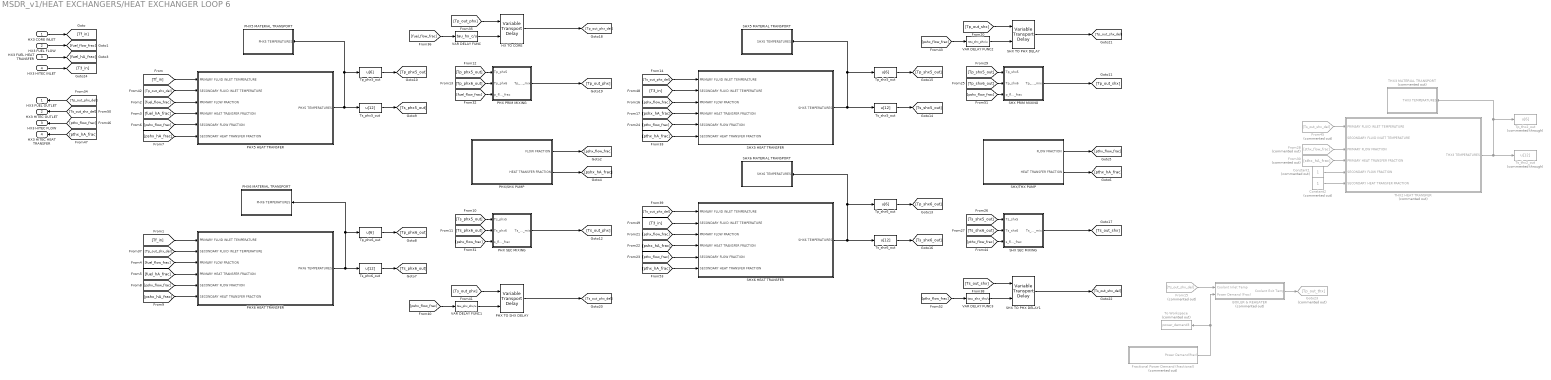
== system MSDR_v1/HEAT EXCHANGERS/HEAT EXCHANGER LOOP 6 ==
  HX3 CORE INLET : Inport
  HX3 FUEL FLOW : Inport  Port=2
  HX3 FUEL HEAT TRANSFER : Inport  Port=3
  HX3 HITEC INLET : Inport  Port=4
  BOILER & REHEATER : Subsystem  Commented=on
  Constant1 : Constant  Commented=on
  Constant2 : Constant  Commented=on
  Fractional Power Demand (fractional) : Subsystem  Commented=on
  From15 : From  Commented=on  GotoTag=Ts_out_shx_del
  From28 : From  Commented=on  GotoTag=sthx_flow_frac
  From30 : From  Commented=on  GotoTag=sthx_hA_frac
  From45 : From  Commented=on  GotoTag=Ts_out_shx_del
  Goto23 : Goto  Commented=on  GotoTag=Tp_out_thx
  HX TO CORE : VariableTransportDelay  MaximumDelay=1000000000000  InitialOutput=T0_p_phx5(4)
  PHX PRIM MIXING : Subsystem
  PHX SEC MIXING : Subsystem
  PHX TO SHX DELAY : VariableTransportDelay  MaximumDelay=100000000000  InitialOutput=T0_s_phx5(4)
  PHX/SHX PUMP : Subsystem
  PHX5 HEAT TRANSFER : Subsystem
  PHX5 MATERIAL TRANSPORT : Subsystem
  PHX6 HEAT TRANSFER : Subsystem
  PHX6 MATERIAL TRANSPORT : Subsystem
  SHX PRIM MIXING : Subsystem
  SHX SEC MIXING : Subsystem
  SHX TO PHX DELAY : VariableTransportDelay  MaximumDelay=1000000000000  InitialOutput=T0_p_shx5(4)
  SHX TO PHX DELAY1 : VariableTransportDelay  MaximumDelay=1000000000000  InitialOutput=T0_s_shx5(4)
  SHX/THX PUMP : Subsystem
  SHX5 HEAT TRANSFER : Subsystem
  SHX5 MATERIAL TRANSPORT : Subsystem
  SHX6 HEAT TRANSFER : Subsystem
  SHX6 MATERIAL TRANSPORT : Subsystem
  THX2 HEAT TRANSFER : Subsystem  Commented=on
  THX3 MATERIAL TRANSPORT : Subsystem  Commented=on
  To Workspace : ToWorkspace  Commented=on  VariableName=power_demand3  SampleTime=-1
  Tp_phx5_out : Fcn  Expr=u[6]
  Tp_phx6_out : Fcn  Expr=u[6]
  Tp_shx5_out : Fcn  Expr=u[6]
  Tp_shx6_out : Fcn  Expr=u[6]
  Tp_thx2_out : Fcn  Commented=through  Expr=u[6]
  Ts_phx5_out : Fcn  Expr=u[12]
  Ts_phx6_out : Fcn  Expr=u[12]
  Ts_shx5_out : Fcn  Expr=u[12]
  Ts_shx6_out : Fcn  Expr=u[12]
  Ts_thx2_out : Fcn  Commented=through  Expr=u[12]
  VAR DELAY FUNC : Fcn  Expr=tau_hx_c/u
  VAR DELAY FUNC1 : Fcn  Expr=tau_phx_shx/u
  VAR DELAY FUNC2 : Fcn  Expr=tau_shx_phx/u
  VAR DELAY FUNC3 : Fcn  Expr=tau_shx_thx/u
  HX3 FUEL OUTLET : Outport
  HX3 HITEC OUTLET : Outport  Port=2
  HX3 HITEC FLOW : Outport  Port=3
  HX3 HITEC HEAT TRANSFER : Outport  Port=4
  wires:
  HX3 FUEL FLOW/1 -> [fuel_flow_frac]
  HX3 FUEL HEAT TRANSFER/1 -> [fuel_hA_frac]
  HX3 CORE INLET/1 -> [Tf_in]
  [Tp_out_phx_del] -> HX3 FUEL OUTLET/1
  PHX5 HEAT TRANSFER/1(PHX5 TEMPERATURES) -> PHX5 MATERIAL TRANSPORT/1(PHX5 TEMPERATURES), Tp_phx5_out/1, Ts_phx5_out/1
  Tp_phx5_out/1 -> [Tp_phx5_out]
  Ts_phx5_out/1 -> [Ts_phx5_out]
  PHX6 HEAT TRANSFER/1(PHX6 TEMPERATURES) -> PHX6 MATERIAL TRANSPORT/1(PHX6 TEMPERATURES), Tp_phx6_out/1, Ts_phx6_out/1
  Tp_phx6_out/1 -> [Tp_phx6_out]
  Ts_phx6_out/1 -> [Ts_phx6_out]
  PHX/SHX PUMP/2(HEAT TRANSFER FRACTION) -> [pshx_hA_frac]
  [pshx_flow_frac] -> PHX SEC MIXING/3(s_flow_frac)
  [Ts_phx5_out] -> PHX SEC MIXING/1(Ts_phx5)
  PHX/SHX PUMP/1(FLOW FRACTION) -> [pshx_flow_frac]
  [Ts_phx6_out] -> PHX SEC MIXING/2(Ts_phx6)
  PHX SEC MIXING/1(Ts_phx_mix) -> [Ts_out_phx]
  [Tp_phx6_out] -> PHX PRIM MIXING/2(Tp_phx6)
  PHX PRIM MIXING/1(Tp_phx_mix) -> [Tp_out_phx]
  [Tp_phx5_out] -> PHX PRIM MIXING/1(Tp_phx5)
  [fuel_flow_frac] -> PHX PRIM MIXING/3(p_flow_frac)
  Ts_shx5_out/1 -> [Ts_shx5_out]
  Tp_shx5_out/1 -> [Tp_shx5_out]
  SHX5 HEAT TRANSFER/1(SHX5 TEMPERATURES) -> Ts_shx5_out/1, SHX5 MATERIAL TRANSPORT/1(SHX5 TEMPERATURES), Tp_shx5_out/1
  SHX6 HEAT TRANSFER/1(SHX6 TEMPERATURES) -> Ts_shx6_out/1, SHX6 MATERIAL TRANSPORT/1(SHX6 TEMPERATURES), Tp_shx6_out/1
  Ts_shx6_out/1 -> [Ts_shx6_out]
  Tp_shx6_out/1 -> [Tp_shx6_out]
  SHX/THX PUMP/1(FLOW FRACTION) -> [pthx_flow_frac]
  SHX SEC MIXING/1(Ts_shx_mix) -> [Ts_out_shx]
  SHX/THX PUMP/2(HEAT TRANSFER FRACTION) -> [pthx_hA_frac]
  SHX PRIM MIXING/1(Tp_shx_mix) -> [Tp_out_shx]
  [Ts_shx5_out] -> SHX SEC MIXING/1(Ts_shx5)
  [Tp_shx5_out] -> SHX PRIM MIXING/1(Tp_shx5)
  [pthx_flow_frac] -> SHX SEC MIXING/3(s_flow_frac)
  [Ts_shx6_out] -> SHX SEC MIXING/2(Ts_shx6)
  [Tp_shx6_out] -> SHX PRIM MIXING/2(Tp_shx6)
  THX2 HEAT TRANSFER/1(THX3 TEMPERATURES) -> THX3 MATERIAL TRANSPORT/1(THX3 TEMPERATURES), Tp_thx2_out/1, Ts_thx2_out/1
  [pshx_hA_frac] -> PHX5 HEAT TRANSFER/6(SECONDARY HEAT TRANSFER FRACTION)
  [Tp_out_shx_del] -> PHX5 HEAT TRANSFER/2(SECONDARY FLUID INLET TEMPERATURE)
  [pshx_flow_frac] -> PHX5 HEAT TRANSFER/5(SECONDARY FLOW FRACTION)
  [fuel_hA_frac] -> PHX5 HEAT TRANSFER/4(PRIMARY HEAT TRANSFER FRACTION)
  [Tf_in] -> PHX5 HEAT TRANSFER/1(PRIMARY FLUID INLET TEMPERATURE)
  [fuel_flow_frac] -> PHX5 HEAT TRANSFER/3(PRIMARY FLOW FRACTION)
  [pshx_flow_frac] -> PHX6 HEAT TRANSFER/5(SECONDARY FLOW FRACTION)
  [fuel_hA_frac] -> PHX6 HEAT TRANSFER/4(PRIMARY HEAT TRANSFER FRACTION)
  [pshx_hA_frac] -> PHX6 HEAT TRANSFER/6(SECONDARY HEAT TRANSFER FRACTION)
  [Tf_in] -> PHX6 HEAT TRANSFER/1(PRIMARY FLUID INLET TEMPERATURE)
  [fuel_flow_frac] -> PHX6 HEAT TRANSFER/3(PRIMARY FLOW FRACTION)
  [Tp_out_shx_del] -> PHX6 HEAT TRANSFER/2(SECONDARY FLUID INLET TEMPERATURE)
  [fuel_flow_frac] -> VAR DELAY FUNC/1
  [Tp_out_phx] -> HX TO CORE/1
  HX TO CORE/1 -> [Tp_out_phx_del]
  VAR DELAY FUNC/1 -> HX TO CORE/2
  PHX TO SHX DELAY/1 -> [Ts_out_phx_del]
  [pshx_flow_frac] -> VAR DELAY FUNC1/1
  VAR DELAY FUNC1/1 -> PHX TO SHX DELAY/2
  [Ts_out_phx] -> PHX TO SHX DELAY/1
  [pshx_flow_frac] -> SHX5 HEAT TRANSFER/3(PRIMARY FLOW FRACTION)
  [pshx_hA_frac] -> SHX5 HEAT TRANSFER/4(PRIMARY HEAT TRANSFER FRACTION)
  [pthx_hA_frac] -> SHX5 HEAT TRANSFER/6(SECONDARY HEAT TRANSFER FRACTION)
  [Ts_out_phx_del] -> SHX5 HEAT TRANSFER/1(PRIMARY FLUID INLET TEMPERATURE)
  [pthx_flow_frac] -> SHX5 HEAT TRANSFER/5(SECONDARY FLOW FRACTION)
  [pthx_hA_frac] -> SHX6 HEAT TRANSFER/6(SECONDARY HEAT TRANSFER FRACTION)
  [pshx_hA_frac] -> SHX6 HEAT TRANSFER/4(PRIMARY HEAT TRANSFER FRACTION)
  [pshx_flow_frac] -> SHX6 HEAT TRANSFER/3(PRIMARY FLOW FRACTION)
  [pthx_flow_frac] -> SHX6 HEAT TRANSFER/5(SECONDARY FLOW FRACTION)
  [Ts_out_phx_del] -> SHX6 HEAT TRANSFER/1(PRIMARY FLUID INLET TEMPERATURE)
  VAR DELAY FUNC2/1 -> SHX TO PHX DELAY/2
  [Tp_out_shx] -> SHX TO PHX DELAY/1
  [pshx_flow_frac] -> VAR DELAY FUNC2/1
  SHX TO PHX DELAY/1 -> [Tp_out_shx_del]
  [Ts_out_shx] -> SHX TO PHX DELAY1/1
  SHX TO PHX DELAY1/1 -> [Ts_out_shx_del]
  [pthx_flow_frac] -> VAR DELAY FUNC3/1
  VAR DELAY FUNC3/1 -> SHX TO PHX DELAY1/2
  Constant1/1 -> THX2 HEAT TRANSFER/5(SECONDARY FLOW FRACTION)
  Constant2/1 -> THX2 HEAT TRANSFER/6(SECONDARY HEAT TRANSFER FRACTION)
  From45/1 -> THX2 HEAT TRANSFER/1(PRIMARY FLUID INLET TEMPERATURE)
  From28/1 -> THX2 HEAT TRANSFER/3(PRIMARY FLOW FRACTION)
  From30/1 -> THX2 HEAT TRANSFER/4(PRIMARY HEAT TRANSFER FRACTION)
  BOILER & REHEATER/1(Coolant Exit Temp) -> Goto23/1
  From15/1 -> BOILER & REHEATER/1(Coolant Inlet Temp)
  Fractional Power Demand (fractional)/1(Power Demand(frac)) -> To Workspace/1, BOILER & REHEATER/2(Power Demand (Frac))
  [T3_in] -> SHX5 HEAT TRANSFER/2(SECONDARY FLUID INLET TEMPERATURE)
  [T3_in] -> SHX6 HEAT TRANSFER/2(SECONDARY FLUID INLET TEMPERATURE)
  HX3 HITEC INLET/1 -> [T3_in]
  [Ts_out_shx_del] -> HX3 HITEC OUTLET/1
  [pthx_flow_frac] -> HX3 HITEC FLOW/1
  [pthx_hA_frac] -> HX3 HITEC HEAT TRANSFER/1
  [pshx_flow_frac] -> SHX PRIM MIXING/3(p_flow_frac)

== system MSDR_v1/HEAT EXCHANGERS/PRE BoP MIXING ==
  Tshx1 : Inport
  delay1 : Inport  Port=2
  Tshx2 : Inport  Port=3
  delay2 : Inport  Port=4
  Tshx3 : Inport  Port=5
  delay3 : Inport  Port=6
  Fcn : Fcn  Expr=u[2]*W_31/m_3m*(u[1] - u[7]) + u[4]*W_32/m_3m*(u[3] - u[7]) + u[6]*W_33/m_3m*(u[5] - u[7])
  Integrator : Integrator  InitialCondition=T3_out
  Mux : Mux  Inputs=7
  T3_out : Outport
  wires:
  Tshx1/1 -> Mux/1
  delay1/1 -> Mux/2
  Tshx2/1 -> Mux/3
  delay2/1 -> Mux/4
  Tshx3/1 -> Mux/5
  delay3/1 -> Mux/6
  Mux/1 -> Fcn/1
  Fcn/1 -> Integrator/1
  Integrator/1 -> T3_out/1, Mux/7

== system MSDR_v1/HEAT EXCHANGERS/PRE CORE MIXING ==
  Tphx1 : Inport
  delay1 : Inport  Port=2
  Tphx2 : Inport  Port=3
  delay2 : Inport  Port=4
  Tphx3 : Inport  Port=5
  delay3 : Inport  Port=6
  Fcn : Fcn  Expr=u[2]*W_f1/m_fm*(u[1] - u[7]) + u[4]*W_f2/m_fm*(u[3] - u[7]) + u[6]*W_f3/m_fm*(u[5] - u[7])
  Integrator : Integrator  InitialCondition=Tf_in
  Mux : Mux  Inputs=7
  Tf_out : Outport
  wires:
  Tphx1/1 -> Mux/1
  delay1/1 -> Mux/2
  Tphx2/1 -> Mux/3
  delay2/1 -> Mux/4
  Tphx3/1 -> Mux/5
  delay3/1 -> Mux/6
  Mux/1 -> Fcn/1
  Fcn/1 -> Integrator/1
  Integrator/1 -> Tf_out/1, Mux/7

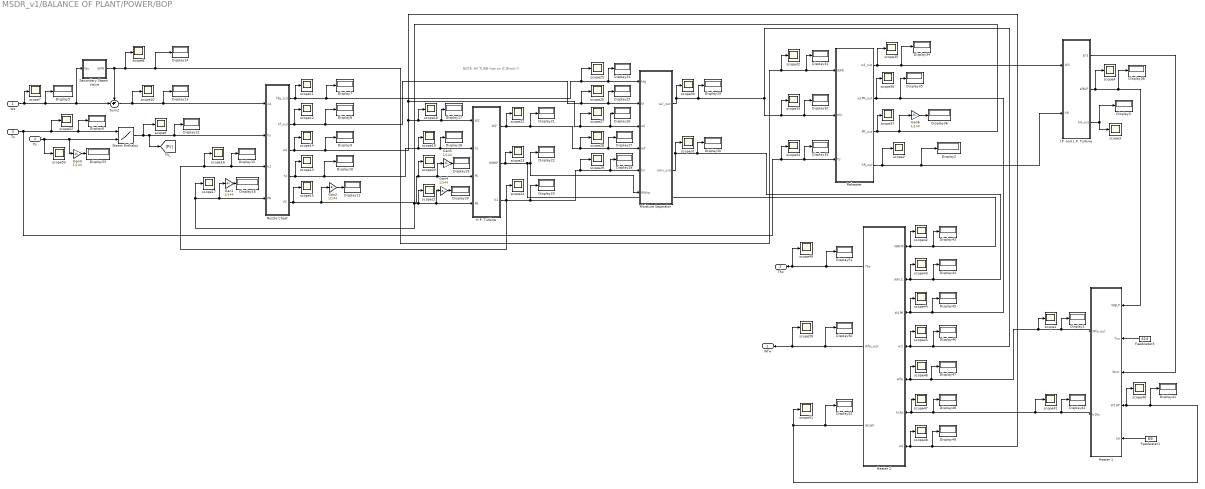
== system MSDR_v1/BALANCE OF PLANT/POWER/BOP ==
  note: NOTE: HP TURB Has an IC Block!!!
  Ws : Inport
  Ps : Inport  Port=2
  Ts : Inport  Port=3
  Display{1..3,5..36,38,41..53} (49 alike) : Display
  Feedwater1 : Constant  Value=69
  Feedwater3 : Constant  Value=414
  Gan{1..6} (6 alike) : Gain  Gain=1/144
  H.P. Turbine : Subsystem
  Heater 1 : Subsystem
  Heater 2 : Subsystem
  I.P. and L.P. Turbine : Subsystem
  Moisture Separator : Subsystem
  Nozzle Chest : Subsystem
  Reheater : Subsystem
  Secondary Steam Valve : Subsystem
  Steam Enthalpy : Lookup_n-D  BreakpointsForDimension1=[550,600,650]  BreakpointsForDimension2=[86400,100800,115200,144000,180000,216000]  Table=[1255.9,1243.8,1230.5,1199.2,1170,1150;1289.9,1280.7,1270.9,1249.3,1217.2,1175.4;1321.3,1313.8,1306.0,1289.5,1266.3,1239.7]  DiagnosticForOutOfRangeInput=Warning  InternalRulePriority=Speed  RndMeth=Simplest  InputSameDT=on
  Sum2 : Sum  Inputs=-+|
  scope{1..4,7..37,40..53} (49 alike) : Scope
  Wfw : Outport
  Tfw : Outport  Port=2
  wires:
  H.P. Turbine/3(h2) -> scope24/1, Display23/1, scope29/1, Display28/1, Moisture Separator/5(h2), scope16/1, Display15/1, Nozzle Chest/3(h2)
  Moisture Separator/1(w2'_out) -> scope30/1, Display29/1, scope33/1, Display32/1, Reheater/2(W2'), Display46/1, scope45/1, Heater 2/4(w'2)
  H.P. Turbine/1(W2'') -> scope22/1, Display21/1, scope28/1, Display27/1, Moisture Separator/4(w2'')
  Secondary Steam Valve/1(WPR) -> Sum2/1, scope32/1, Display31/1, Reheater/1(WPR), Display14/1, scope8/1
  Reheater/3(PR_out) -> scope37/1, Gan6/1, scope21/1, H.P. Turbine/4(PR), Gan4/1, Nozzle Chest/4(PR), Gan1/1, scope17/1
  Heater 1/1(Wfw_out) -> Display1/1, scope1/1, Display47/1, scope46/1, Heater 2/5(Wfw)
  Heater 1/2(h1fw) -> Display42/1, scope41/1, Display48/1, scope47/1, Heater 2/6(h1fw)
  Reheater/1(w3_out) -> scope35/1, I.P. and L.P. Turbine/1(W3), Display34/1
  Moisture Separator/2(wms_out) -> scope31/1, Display30/1, Display44/1, scope43/1, Heater 2/2(WM.S.)
  Reheater/2(w1PR_out) -> scope36/1, Display45/1, scope44/1, Heater 2/3(W1PR), Display35/1
  H.P. Turbine/2(WBHP) -> scope23/1, Moisture Separator/6(Wbhp), Display22/1, Display43/1, scope42/1, Heater 2/1(WBHP)
  Ps/1 -> Gan3/1, Steam Enthalpy/2, scope53/1
  Nozzle Chest/2(hf_out) -> scope12/1, Display8/1, scope26/1, Display25/1, Moisture Separator/2(hf)
  Nozzle Chest/4(hc) -> scope13/1, Display10/1, scope19/1, Display18/1, H.P. Turbine/2(hc)
  Nozzle Chest/3(w2) -> scope14/1, Display9/1, Display49/1, scope48/1, Heater 2/7(w2), scope27/1, Display26/1, Moisture Separator/3(w2), scope18/1, Display17/1, H.P. Turbine/1(W2)
  Ws/1 -> scope7/1, Display5/1, Sum2/2, Secondary Steam Valve/1(Ws)
  Sum2/1 -> scope10/1, Display13/1, Nozzle Chest/1(w1)
  I.P. and L.P. Turbine/1(W'3) -> Heater 1/3(Wco')
  Ts/1 -> scope52/1, Display6/1, Steam Enthalpy/1, scope34/1, Display33/1, Reheater/3(Ts)
  Steam Enthalpy/1 -> scope9/1, [Ps], Nozzle Chest/2(hs), Display12/1
  Heater 2/2(Wfw_out) -> Display50/1, Wfw/1, scope50/1
  Heater 2/3(W1HP) -> Display52/1, scope51/1, Display41/1, scope40/1, Heater 1/4(W1HP)
  I.P. and L.P. Turbine/2(WBLP) -> scope4/1, Heater 1/1(WBLP), Display38/1
  Nozzle Chest/5(PC) -> scope15/1, scope20/1, H.P. Turbine/3(PC), Gan5/1, Gan2/1
  Nozzle Chest/1(hfg_out) -> scope11/1, Display7/1, scope25/1, Display24/1, Moisture Separator/1(hfg)
  Gan2/1 -> Display11/1
  Gan1/1 -> Display16/1
  Gan3/1 -> Display53/1
  Gan5/1 -> Display19/1
  Gan4/1 -> Display20/1
  Gan6/1 -> Display36/1
  Heater 2/1(Tfw) -> Display51/1, Tfw/1, scope49/1
  Feedwater3/1 -> Heater 1/2(Tco)
  Reheater/4(hR_out) -> scope2/1, Display2/1, I.P. and L.P. Turbine/2(hR)
  I.P. and L.P. Turbine/3(h4_out) -> scope3/1, Display3/1
  Feedwater1/1 -> Heater 1/5(h0)
